simulink model "Control_RawPitchYaw"  (R2015b)
settings: Solver=FixedStepDiscrete  StartTime=0.0  StopTime=inf  FixedStep=0.03  RelTol=1e-3
undefined symbols (not defined in the file): DiscIntNeverNeededParam
libraries: simulink x7, arduinolib x4, RASPlib x2
settings Model: SimulationMode=external  ExtModeTrigDuration=2  Creator=jorge  LastModifiedBy=Emilio
settings OptimizationCC: OptimizeModelRefInitCode=on  LifeSpan=Inf  MaxStackSize=64
settings HardwareCC: ProdBitPerInt=16  ProdBitPerPointer=16  ProdLargestAtomicFloat=None  ProdWordSize=8  ProdHWDeviceType=Atmel->AVR
settings RTWCC: SystemTargetFile=ert.tlc  TemplateMakefile=ert_default_tmf  Description=Embedded Coder  Toolchain=Arduino AVR v1.6.1  BuildConfiguration=Faster Runs
settings CodeAppCC: IgnoreCustomStorageClasses=off
settings ERTTargetCC: SupportContinuousTime=on  SupportVariableSizeSignals=on  ExtMode=on  ExtModeMexFile=ext_serial_win32_comm_rtt  ExtModeMexArgs=0 5 115200

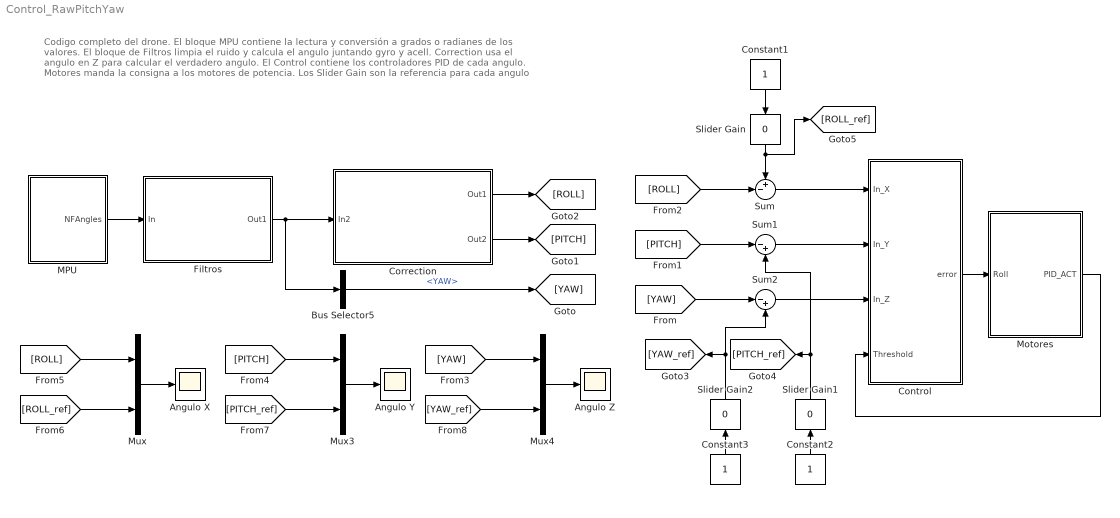
== system Control_RawPitchYaw ==
  note: Codigo completo del drone.
      | El bloque MPU contiene la lectura y conversión a grados o radianes de los valores.
      | El bloque de Filtros limpia el ruido y calcula el angulo juntando gyro y acell.
      | Correction usa el angulo en Z para calcular el verdadero angulo.
      | El Control contiene los controladores PID de cada angulo.
      | Motores manda la consigna a los motores de potencia.
      | Los Slider Gain son la referencia para cada angulo
  Angulo X : Scope
  Angulo Y : Scope
  Angulo Z : Scope
  Bus Selector5 : BusSelector  OutputSignals=YAW
  Constant1 : Constant
  Constant2 : Constant
  Constant3 : Constant
  Control : Subsystem
  Correction : Subsystem
  Filtros : Subsystem
  "MPU " : Subsystem
  "Motores " : Subsystem
  Mux : Mux  Inputs=2
  Mux3 : Mux  Inputs=2
  Mux4 : Mux  Inputs=2
  Slider Gain : simulink/Math Operations/Slider Gain  low=-25  gain=0  high=35
  Slider Gain1 : simulink/Math Operations/Slider Gain  low=-25  gain=0  high=35
  Slider Gain2 : simulink/Math Operations/Slider Gain  low=-25  gain=0  high=35
  Sum : Sum  Inputs=+-|
  Sum1 : Sum  Inputs=|-+
  Sum2 : Sum  Inputs=|-+
  wires:
  Mux/1 -> Angulo X/1
  Constant1/1 -> Slider Gain/1
  Slider Gain/1 -> Sum/1, [ROLL_ref]
  Constant2/1 -> Slider Gain1/1
  Sum/1 -> Control/1(In_X)
  Sum1/1 -> Control/2(In_Y)
  "Motores "/1(PID_ACT) -> Control/4(Threshold)
  Constant3/1 -> Slider Gain2/1
  Slider Gain2/1 -> Sum2/2, [YAW_ref]
  Sum2/1 -> Control/3(In_Z)
  Filtros/1(Out1) -> Bus Selector5/1, Correction/1(In2)
  "MPU "/1(NFAngles) -> Filtros/1(In)
  Bus Selector5/1 -> [YAW]  "<YAW>"
  Correction/2(Out2) -> [PITCH]
  Correction/1(Out1) -> [ROLL]
  [YAW] -> Sum2/1
  [PITCH] -> Sum1/1
  [ROLL] -> Sum/2
  Slider Gain1/1 -> [PITCH_ref], Sum1/2
  [ROLL] -> Mux/1
  [ROLL_ref] -> Mux/2
  [PITCH] -> Mux3/1
  [YAW] -> Mux4/1
  Mux3/1 -> Angulo Y/1
  Mux4/1 -> Angulo Z/1
  [PITCH_ref] -> Mux3/2
  [YAW_ref] -> Mux4/2
  Control/1(error) -> "Motores "/1(Roll)

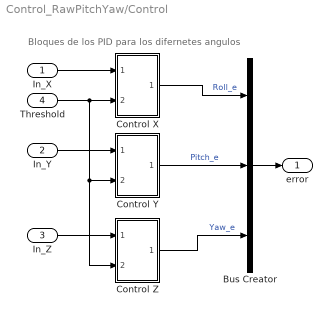
== system Control_RawPitchYaw/Control ==
  note: Bloques de los PID para los difernetes angulos
  In_X : Inport
  In_Y : Inport  Port=2
  In_Z : Inport  Port=3
  Threshold : Inport  Port=4
  Bus Creator : BusCreator  Inputs=3
  Control X : Subsystem
  Control Y : Subsystem
  Control Z : Subsystem
  error : Outport
  wires:
  Control X/1(Out1) -> Bus Creator/1  "Roll_e"
  Control Y/1(Out1) -> Bus Creator/2  "Pitch_e"
  In_Y/1 -> Control Y/1(In1)
  In_X/1 -> Control X/1(In1)
  In_Z/1 -> Control Z/1(In1)
  Threshold/1 -> Control Z/2(Threshold), Control Y/2(Threshold), Control X/2(Threshold)
  Control Z/1(Out1) -> Bus Creator/3  "Yaw_e"
  Bus Creator/1 -> error/1

== system Control_RawPitchYaw/Correction ==
  In2 : Inport
  Bus Selector3 : BusSelector  OutputSignals=NCAngle_X,NCAngle_y,Angle_Zrad
  Bus Selector4 : BusSelector  OutputSignals=NCAngle_y,NCAngle_X,Angle_Zrad
  CorrectionPITCH : Subsystem
  CorrectionROLL : Subsystem
  Out1 : Outport
  Out2 : Outport  Port=2
  wires:
  In2/1 -> Bus Selector3/1, Bus Selector4/1
  Bus Selector4/2 -> CorrectionPITCH/2(Angle_Corr)  "<NCAngle_X>"
  Bus Selector3/1 -> CorrectionROLL/1(Angle_cal)  "<NCAngle_X>"
  Bus Selector3/3 -> CorrectionROLL/3(Z_Corr)  "<Angle_Zrad>"
  Bus Selector4/1 -> CorrectionPITCH/1(Angle_cal)  "<NCAngle_y>"
  Bus Selector3/2 -> CorrectionROLL/2(Angle_Corr)  "<NCAngle_y>"
  Bus Selector4/3 -> CorrectionPITCH/3(Z_Corr)  "<Angle_Zrad>"
  CorrectionPITCH/1(Angle_Corrected) -> Out2/1  "PITCH"
  CorrectionROLL/1(Angle_Corrected) -> Out1/1  "ROLL"

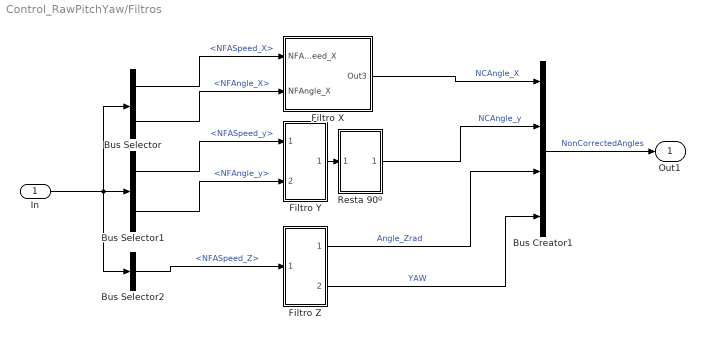
== system Control_RawPitchYaw/Filtros ==
  In : Inport
  Bus Creator1 : BusCreator  Inputs=4
  Bus Selector : BusSelector  OutputSignals=NFASpeed_X,NFAngle_X
  Bus Selector1 : BusSelector  OutputSignals=NFASpeed_y,NFAngle_y
  Bus Selector2 : BusSelector  OutputSignals=NFASpeed_Z
  Filtro X : Subsystem
  Filtro Y : Subsystem
  "Filtro Z " : Subsystem
  Resta 90º : Subsystem
  Out1 : Outport
  wires:
  Bus Creator1/1 -> Out1/1  "NonCorrectedAngles"
  Filtro X/1(Out3) -> Bus Creator1/1  "NCAngle_X"
  Bus Selector/1 -> Filtro X/1(NFASpeed_X)  "<NFASpeed_X>"
  Bus Selector2/1 -> "Filtro Z "/1(In1)  "<NFASpeed_Z>"
  Bus Selector1/1 -> Filtro Y/1(In1)  "<NFASpeed_y>"
  Bus Selector/2 -> Filtro X/2(NFAngle_X)  "<NFAngle_X>"
  Bus Selector1/2 -> Filtro Y/2(In2)  "<NFAngle_y>"
  In/1 -> Bus Selector/1, Bus Selector2/1, Bus Selector1/1
  Resta 90º/1(Out1) -> Bus Creator1/2  "NCAngle_y"
  "Filtro Z "/1(Z radianes) -> Bus Creator1/3  "Angle_Zrad"
  Filtro Y/1(Out3) -> Resta 90º/1(In1)
  "Filtro Z "/2(Z grados) -> Bus Creator1/4  "YAW"

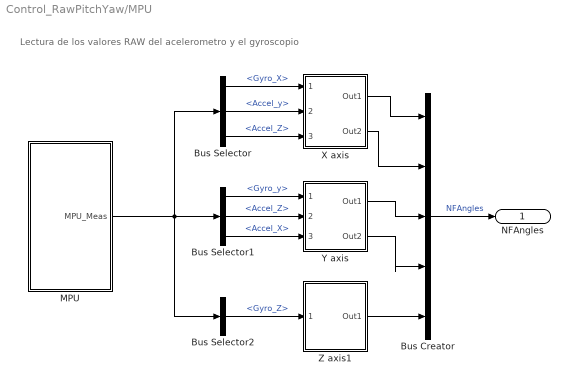
== system Control_RawPitchYaw/MPU  ==
  note: Lectura de los valores RAW del acelerometro y el gyroscopio
  Bus Creator : BusCreator  Inputs='NFASpeed_X','NFAngle_X','NFASpeed_y','NFAngle_y','NFASpeed_Z'
  Bus Selector : BusSelector  OutputSignals=Gyro_X,Accel_y,Accel_Z
  Bus Selector1 : BusSelector  OutputSignals=Gyro_y,Accel_Z,Accel_X
  Bus Selector2 : BusSelector  OutputSignals=Gyro_Z
  MPU : Subsystem
  X axis : Subsystem
  Y axis : Subsystem
  Z axis1 : Subsystem
  NFAngles : Outport
  wires:
  MPU/1(MPU_Meas) -> Bus Selector/1, Bus Selector1/1, Bus Selector2/1
  Bus Selector/2 -> X axis/2(Accel_y)  "<Accel_y>"
  Bus Selector/3 -> X axis/3(Accel_Z)  "<Accel_Z>"
  Bus Selector/1 -> X axis/1(Gyro_X)  "<Gyro_X>"
  Bus Selector1/2 -> Y axis/2(Accel_Z)  "<Accel_Z>"
  Bus Selector1/3 -> Y axis/3(Accel_X)  "<Accel_X>"
  Bus Selector1/1 -> Y axis/1(Gyro_y)  "<Gyro_y>"
  Bus Selector2/1 -> Z axis1/1(Gyro_Z)  "<Gyro_Z>"
  Bus Creator/1 -> NFAngles/1  "NFAngles"
  X axis/1(Out1) -> Bus Creator/1
  X axis/2(Out2) -> Bus Creator/2
  Y axis/1(Out1) -> Bus Creator/3
  Y axis/2(Out2) -> Bus Creator/4
  Z axis1/1(Out1) -> Bus Creator/5

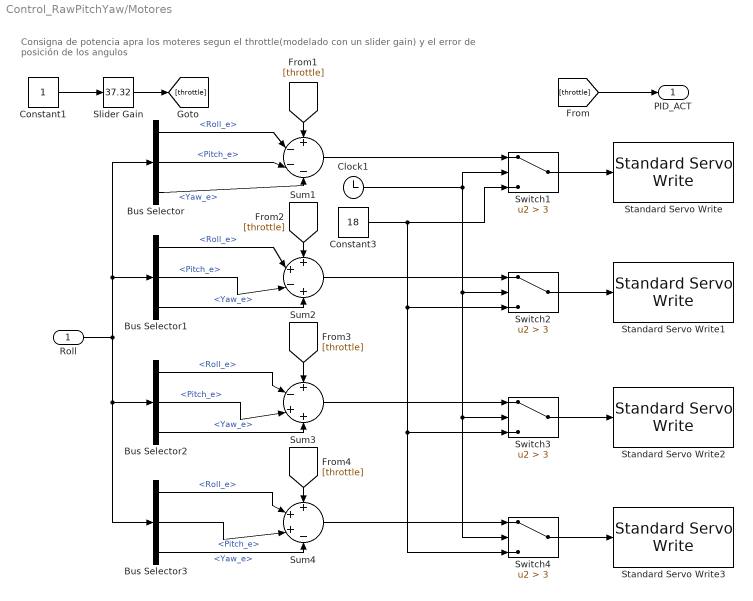
== system Control_RawPitchYaw/Motores  ==
  note: Consigna de potencia apra los moteres segun el throttle(modelado con un slider gain) y el error de posición de los angulos
  Roll : Inport
  Bus Selector{,1..3} (4 alike) : BusSelector  OutputSignals=Roll_e,Pitch_e,Yaw_e
  Clock1 : Clock
  Constant1 : Constant
  Constant3 : Constant  Value=18
  Slider Gain : simulink/Math Operations/Slider Gain  low=18  gain=37.32  high=60
  Standard Servo Write : arduinolib/Standard Servo Write  pinNumber=12  blockPlatform=arduino
  Standard Servo Write1 : arduinolib/Standard Servo Write  pinNumber=11  blockPlatform=arduino
  Standard Servo Write2 : arduinolib/Standard Servo Write  pinNumber=10  blockPlatform=arduino
  Standard Servo Write3 : arduinolib/Standard Servo Write  pinNumber=9  blockPlatform=arduino
  Sum1 : Sum  Inputs=+|-|-|-
  Sum2 : Sum  Inputs=+|+|-|+
  Sum3 : Sum  Inputs=+|-|+|+
  Sum4 : Sum  Inputs=+|+|+|-
  Switch{1..4} (4 alike) : Switch  Criteria=u2 > Threshold  Threshold=3
  PID_ACT : Outport
  wires:
  Constant3/1 -> Switch4/3, Switch3/3, Switch2/3, Switch1/3
  Sum4/1 -> Switch4/1
  Clock1/1 -> Switch1/2, Switch4/2, Switch3/2, Switch2/2
  Sum3/1 -> Switch3/1
  Switch4/1 -> Standard Servo Write3/1
  Switch3/1 -> Standard Servo Write2/1
  Sum1/1 -> Switch1/1
  Switch1/1 -> Standard Servo Write/1
  Switch2/1 -> Standard Servo Write1/1
  Sum2/1 -> Switch2/1
  Constant1/1 -> Slider Gain/1
  Roll/1 -> Bus Selector3/1, Bus Selector2/1, Bus Selector/1, Bus Selector1/1
  Bus Selector/1 -> Sum1/2  "<Roll_e>"
  Bus Selector/2 -> Sum1/3  "<Pitch_e>"
  Bus Selector/3 -> Sum1/4  "<Yaw_e>"
  Bus Selector1/1 -> Sum2/2  "<Roll_e>"
  Bus Selector1/2 -> Sum2/3  "<Pitch_e>"
  Bus Selector1/3 -> Sum2/4  "<Yaw_e>"
  Bus Selector2/1 -> Sum3/2  "<Roll_e>"
  Bus Selector2/2 -> Sum3/3  "<Pitch_e>"
  Bus Selector2/3 -> Sum3/4  "<Yaw_e>"
  Bus Selector3/1 -> Sum4/2  "<Roll_e>"
  Bus Selector3/2 -> Sum4/3  "<Pitch_e>"
  Bus Selector3/3 -> Sum4/4  "<Yaw_e>"
  Slider Gain/1 -> [throttle]
  [throttle] -> PID_ACT/1
  [throttle] -> Sum1/1
  [throttle] -> Sum2/1
  [throttle] -> Sum3/1
  [throttle] -> Sum4/1

== system Control_RawPitchYaw/Control/Control X ==
  note: PID con un threshold apra evitar que el integrador acumule antes que el control pueda mover el drone
  In1 : Inport
  Threshold : Inport  Port=2
  Constant2 : Constant  Value=0
  Discrete PID Controller : simulink/Continuous/PID Controller  Controller=PID  TimeDomain=Discrete-time  SampleTime=-1  IntegratorMethod=Forward Euler  FilterMethod=Forward Euler  Form=Parallel  UseFilter=off  ControllerParametersSource=internal  P=0.51  I=0.43  D=0.15  N=30  InitialConditionSource=internal  InitialConditionForIntegrator=0  InitialConditionForFilter=0  ExternalReset=rising  LimitOutput=off  UpperSaturationLimit=inf  LowerSaturationLimit=-inf  LinearizeAsGain=off  AntiWindupMode=none  Kb=1  TrackingMode=off  Kt=1  PParamMin=[]  PParamMax=[]  IParamMin=[]  IParamMax=[]  DParamMin=[]  DParamMax=[]  NParamMin=[]  NParamMax=[]  KbParamMin=[]  KbParamMax=[]  KtParamMin=[]  KtParamMax=[]  POutMin=[]  POutMax=[]  IOutMin=[]  IOutMax=[]  DOutMin=[]  DOutMax=[]  NOutMin=[]  NOutMax=[]  KbOutMin=[]  KbOutMax=[]  KtOutMin=[]  KtOutMax=[]  IntegratorOutMin=[]  IntegratorOutMax=[]  FilterOutMin=[]  FilterOutMax=[]  SumOutMin=[]  SumOutMax=[]  SumI1OutMin=[]  SumI1OutMax=[]  SumI2OutMin=[]  SumI2OutMax=[]  SumI3OutMin=[]  SumI3OutMax=[]  SumDOutMin=[]  SumDOutMax=[]  SaturationOutMin=[]  SaturationOutMax=[]  IntegratorContinuousStateAttributes=''  IntegratorStateMustResolveToSignalObject=off  IntegratorRTWStateStorageClass=Auto  FilterContinuousStateAttributes=''  FilterStateMustResolveToSignalObject=off  FilterRTWStateStorageClass=Auto  DifferentiatorICPrevScaledInput=0  DifferentiatorOutMin=[]  DifferentiatorOutMax=[]
  Pulse Generator : DiscretePulseGenerator  Commented=on  Period=167  PulseWidth=5  SampleTime=0.03
  Switch1 : Switch  Criteria=u2 > Threshold  Threshold=35
  Out1 : Outport
  wires:
  Discrete PID Controller/1 -> Out1/1
  Switch1/1 -> Discrete PID Controller/1
  Threshold/1 -> Switch1/2
  Constant2/1 -> Switch1/3
  In1/1 -> Switch1/1
  Pulse Generator/1 -> Discrete PID Controller/2

== system Control_RawPitchYaw/Control/Control Y ==
  In1 : Inport
  Threshold : Inport  Port=2
  Constant2 : Constant  Value=0
  Discrete PID Controller : simulink/Continuous/PID Controller  Controller=PID  TimeDomain=Discrete-time  SampleTime=-1  IntegratorMethod=Forward Euler  FilterMethod=Forward Euler  Form=Parallel  UseFilter=off  ControllerParametersSource=internal  P=0.51  I=0.43  D=0.15  N=30  InitialConditionSource=internal  InitialConditionForIntegrator=0  InitialConditionForFilter=0  ExternalReset=rising  LimitOutput=off  UpperSaturationLimit=inf  LowerSaturationLimit=-inf  LinearizeAsGain=off  AntiWindupMode=none  Kb=1  TrackingMode=off  Kt=1  PParamMin=[]  PParamMax=[]  IParamMin=[]  IParamMax=[]  DParamMin=[]  DParamMax=[]  NParamMin=[]  NParamMax=[]  KbParamMin=[]  KbParamMax=[]  KtParamMin=[]  KtParamMax=[]  POutMin=[]  POutMax=[]  IOutMin=[]  IOutMax=[]  DOutMin=[]  DOutMax=[]  NOutMin=[]  NOutMax=[]  KbOutMin=[]  KbOutMax=[]  KtOutMin=[]  KtOutMax=[]  IntegratorOutMin=[]  IntegratorOutMax=[]  FilterOutMin=[]  FilterOutMax=[]  SumOutMin=[]  SumOutMax=[]  SumI1OutMin=[]  SumI1OutMax=[]  SumI2OutMin=[]  SumI2OutMax=[]  SumI3OutMin=[]  SumI3OutMax=[]  SumDOutMin=[]  SumDOutMax=[]  SaturationOutMin=[]  SaturationOutMax=[]  IntegratorContinuousStateAttributes=''  IntegratorStateMustResolveToSignalObject=off  IntegratorRTWStateStorageClass=Auto  FilterContinuousStateAttributes=''  FilterStateMustResolveToSignalObject=off  FilterRTWStateStorageClass=Auto  DifferentiatorICPrevScaledInput=0  DifferentiatorOutMin=[]  DifferentiatorOutMax=[]
  Pulse Generator : DiscretePulseGenerator  Commented=on  Period=167  PulseWidth=5  SampleTime=0.03
  Switch1 : Switch  Criteria=u2 > Threshold  Threshold=35
  Out1 : Outport
  wires:
  Discrete PID Controller/1 -> Out1/1
  Switch1/1 -> Discrete PID Controller/1
  Threshold/1 -> Switch1/2
  Constant2/1 -> Switch1/3
  In1/1 -> Switch1/1
  Pulse Generator/1 -> Discrete PID Controller/2

== system Control_RawPitchYaw/Control/Control Z ==
  In1 : Inport
  Threshold : Inport  Port=2
  Constant2 : Constant  Value=0
  Discrete PID Controller : simulink/Continuous/PID Controller  Controller=PID  TimeDomain=Discrete-time  SampleTime=-1  IntegratorMethod=Forward Euler  FilterMethod=Forward Euler  Form=Parallel  UseFilter=off  ControllerParametersSource=internal  P=0.1  I=0  D=0  N=30  InitialConditionSource=internal  InitialConditionForIntegrator=0  InitialConditionForFilter=0  ExternalReset=rising  LimitOutput=off  UpperSaturationLimit=inf  LowerSaturationLimit=-inf  LinearizeAsGain=off  AntiWindupMode=none  Kb=1  TrackingMode=off  Kt=1  PParamMin=[]  PParamMax=[]  IParamMin=[]  IParamMax=[]  DParamMin=[]  DParamMax=[]  NParamMin=[]  NParamMax=[]  KbParamMin=[]  KbParamMax=[]  KtParamMin=[]  KtParamMax=[]  POutMin=[]  POutMax=[]  IOutMin=[]  IOutMax=[]  DOutMin=[]  DOutMax=[]  NOutMin=[]  NOutMax=[]  KbOutMin=[]  KbOutMax=[]  KtOutMin=[]  KtOutMax=[]  IntegratorOutMin=[]  IntegratorOutMax=[]  FilterOutMin=[]  FilterOutMax=[]  SumOutMin=[]  SumOutMax=[]  SumI1OutMin=[]  SumI1OutMax=[]  SumI2OutMin=[]  SumI2OutMax=[]  SumI3OutMin=[]  SumI3OutMax=[]  SumDOutMin=[]  SumDOutMax=[]  SaturationOutMin=[]  SaturationOutMax=[]  IntegratorContinuousStateAttributes=''  IntegratorStateMustResolveToSignalObject=off  IntegratorRTWStateStorageClass=Auto  FilterContinuousStateAttributes=''  FilterStateMustResolveToSignalObject=off  FilterRTWStateStorageClass=Auto  DifferentiatorICPrevScaledInput=0  DifferentiatorOutMin=[]  DifferentiatorOutMax=[]
  Pulse Generator : DiscretePulseGenerator  Commented=on  Period=167  PulseWidth=5  SampleTime=0.03
  Switch1 : Switch  Criteria=u2 > Threshold  Threshold=25
  Out1 : Outport
  wires:
  Discrete PID Controller/1 -> Out1/1
  Switch1/1 -> Discrete PID Controller/1
  Threshold/1 -> Switch1/2
  Constant2/1 -> Switch1/3
  In1/1 -> Switch1/1
  Pulse Generator/1 -> Discrete PID Controller/2

== system Control_RawPitchYaw/Correction/CorrectionPITCH ==
  note: Correción al angulo usando las medidas en Z
  Angle_cal : Inport
  Angle_Corr : Inport  Port=2
  Z_Corr : Inport  Port=3
  Product : Product
  Sum2 : Sum  Inputs=++|
  Trigonometric Function : Trigonometry
  Angle_Corrected : Outport
  wires:
  Angle_Corr/1 -> Product/1
  Sum2/1 -> Angle_Corrected/1
  Z_Corr/1 -> Trigonometric Function/1
  Angle_cal/1 -> Sum2/1
  Product/1 -> Sum2/2
  Trigonometric Function/1 -> Product/2

== system Control_RawPitchYaw/Correction/CorrectionROLL ==
  note: Correción al angulo usando las medidas en Z
  Angle_cal : Inport
  Angle_Corr : Inport  Port=2
  Z_Corr : Inport  Port=3
  Product : Product
  Sum2 : Sum  Inputs=++|
  Trigonometric Function : Trigonometry
  Angle_Corrected : Outport
  wires:
  Trigonometric Function/1 -> Product/2
  Product/1 -> Sum2/2
  Angle_cal/1 -> Sum2/1
  Z_Corr/1 -> Trigonometric Function/1
  Sum2/1 -> Angle_Corrected/1
  Angle_Corr/1 -> Product/1

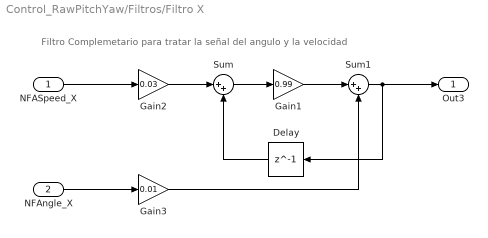
== system Control_RawPitchYaw/Filtros/Filtro X ==
  note: Filtro Complemetario para tratar la señal del angulo y la velocidad
  NFASpeed_X : Inport
  NFAngle_X : Inport  Port=2
  Delay : Delay  DelayLength=1  InitialCondition=0
  Gain1 : Gain  Gain=0.99
  Gain2 : Gain  Gain=0.03
  Gain3 : Gain  Gain=0.01
  Sum : Sum  Inputs=|++
  Sum1 : Sum  Inputs=|++
  Out3 : Outport
  wires:
  Delay/1 -> Sum/2
  Sum/1 -> Gain1/1
  NFAngle_X/1 -> Gain3/1
  Gain1/1 -> Sum1/1
  Sum1/1 -> Out3/1, Delay/1
  NFASpeed_X/1 -> Gain2/1
  Gain2/1 -> Sum/1
  Gain3/1 -> Sum1/2

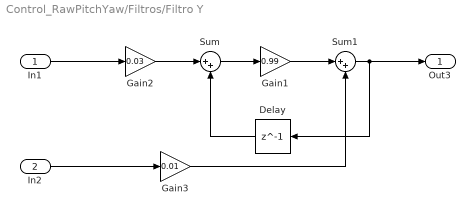
== system Control_RawPitchYaw/Filtros/Filtro Y ==
  In1 : Inport
  In2 : Inport  Port=2
  Delay : Delay  DelayLength=1  InitialCondition=0
  Gain1 : Gain  Gain=0.99
  Gain2 : Gain  Gain=0.03
  Gain3 : Gain  Gain=0.01
  Sum : Sum  Inputs=|++
  Sum1 : Sum  Inputs=|++
  Out3 : Outport
  wires:
  Delay/1 -> Sum/2
  Sum/1 -> Gain1/1
  In2/1 -> Gain3/1
  Gain1/1 -> Sum1/1
  Sum1/1 -> Out3/1, Delay/1
  In1/1 -> Gain2/1
  Gain2/1 -> Sum/1
  Gain3/1 -> Sum1/2

== system Control_RawPitchYaw/Filtros/Filtro Z  ==
  note: Integración de la velocidad en Z para sacar el angulo en radianes y grados
  In1 : Inport
  Discrete-Time Integrator : DiscreteIntegrator  InitialConditionSetting=State (most efficient)  SampleTime=-1  ICPrevOutput=DiscIntNeverNeededParam  ICPrevScaledInput=DiscIntNeverNeededParam
  Gain : Gain  Gain=3.1416/180
  Z radianes : Outport
  Z grados : Outport  Port=2
  wires:
  In1/1 -> Discrete-Time Integrator/1
  Gain/1 -> Z radianes/1
  Discrete-Time Integrator/1 -> Z grados/1, Gain/1

== system Control_RawPitchYaw/Filtros/Resta 90º ==
  In1 : Inport
  Add : Sum  Inputs=+-
  resta90º : Constant  Value=90
  Out1 : Outport
  wires:
  resta90º/1 -> Add/2
  In1/1 -> Add/1
  Add/1 -> Out1/1

== system Control_RawPitchYaw/MPU /MPU ==
  note: Valores RAW de los sensores
  Accelerometer : RASPlib/Accelerometer  SimulateUsing=Code generation
  Bus Creator : BusCreator  Inputs='Gyro_X','Gyro_y','Gyro_Z','Accel_X','Accel_y','Accel_Z'
  Gyroscope : RASPlib/Gyroscope  DLPFmode=0
  MPU_Meas : Outport
  wires:
  Accelerometer/3 -> Bus Creator/6  "Accel_Z"
  Gyroscope/3 -> Bus Creator/3  "Gyro_Z"
  Accelerometer/2 -> Bus Creator/5  "Accel_y"
  Gyroscope/2 -> Bus Creator/2  "Gyro_y"
  Accelerometer/1 -> Bus Creator/4  "Accel_X"
  Bus Creator/1 -> MPU_Meas/1  "MPU_meas"
  Gyroscope/1 -> Bus Creator/1  "Gyro_X"

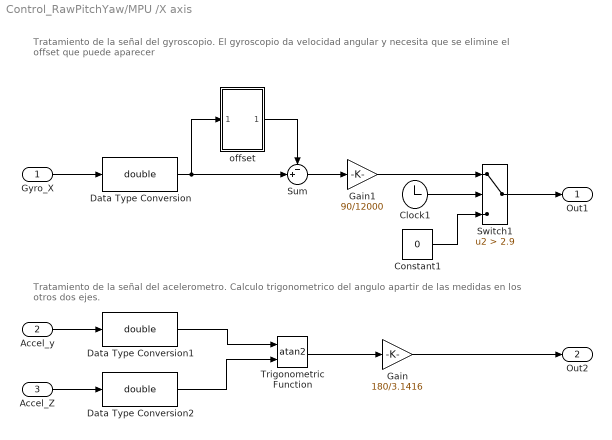
== system Control_RawPitchYaw/MPU /X axis ==
  note: Tratamiento de la señal del acelerometro.
      | Calculo trigonometrico del angulo apartir de las medidas en los otros dos ejes.
  note: Tratamiento de la señal del gyroscopio.
      | El gyroscopio da velocidad angular y necesita que se elimine el offset que puede aparecer
  Gyro_X : Inport
  Accel_y : Inport  Port=2
  Accel_Z : Inport  Port=3
  Clock1 : Clock
  Constant1 : Constant  Value=0
  Data Type Conversion : DataTypeConversion  OutDataTypeStr=double
  Data Type Conversion1 : DataTypeConversion  OutDataTypeStr=double
  Data Type Conversion2 : DataTypeConversion  OutDataTypeStr=double
  Gain : Gain  Gain=180/3.1416
  Gain1 : Gain  Gain=90/12000
  Sum : Sum  Inputs=-+|
  Switch1 : Switch  Criteria=u2 > Threshold  Threshold=2.9
  Trigonometric Function : Trigonometry  Operator=atan2
  offset : Subsystem
  Out1 : Outport
  Out2 : Outport  Port=2
  wires:
  Sum/1 -> Gain1/1
  Gain/1 -> Out2/1
  Clock1/1 -> Switch1/2
  Trigonometric Function/1 -> Gain/1
  Data Type Conversion/1 -> offset/1(In1), Sum/2
  Switch1/1 -> Out1/1
  Data Type Conversion1/1 -> Trigonometric Function/1
  Data Type Conversion2/1 -> Trigonometric Function/2
  Accel_y/1 -> Data Type Conversion1/1
  Constant1/1 -> Switch1/3
  Accel_Z/1 -> Data Type Conversion2/1
  Gyro_X/1 -> Data Type Conversion/1
  Gain1/1 -> Switch1/1
  offset/1(Out1) -> Sum/1

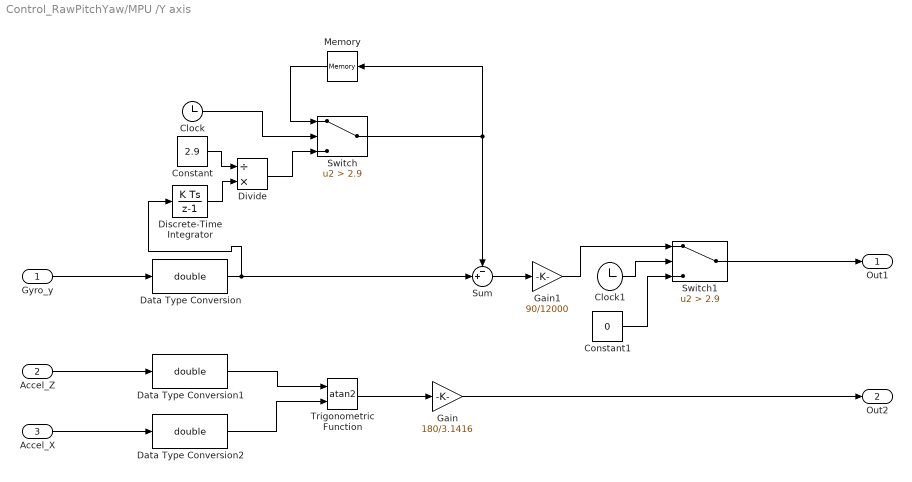
== system Control_RawPitchYaw/MPU /Y axis ==
  Gyro_y : Inport
  Accel_Z : Inport  Port=2
  Accel_X : Inport  Port=3
  Clock : Clock
  Clock1 : Clock
  Constant : Constant  Value=2.9
  Constant1 : Constant  Value=0
  Data Type Conversion : DataTypeConversion  OutDataTypeStr=double
  Data Type Conversion1 : DataTypeConversion  OutDataTypeStr=double
  Data Type Conversion2 : DataTypeConversion  OutDataTypeStr=double
  Discrete-Time Integrator : DiscreteIntegrator  InitialConditionSetting=State (most efficient)  SampleTime=-1  ICPrevOutput=DiscIntNeverNeededParam  ICPrevScaledInput=DiscIntNeverNeededParam
  Divide : Product  Inputs=/*
  Gain : Gain  Gain=180/3.1416
  Gain1 : Gain  Gain=90/12000
  Memory : Memory
  Sum : Sum  Inputs=-+|
  Switch : Switch  Criteria=u2 > Threshold  Threshold=2.9
  Switch1 : Switch  Criteria=u2 > Threshold  Threshold=2.9
  Trigonometric Function : Trigonometry  Operator=atan2
  Out1 : Outport
  Out2 : Outport  Port=2
  wires:
  Sum/1 -> Gain1/1
  Clock/1 -> Switch/2
  Switch/1 -> Sum/1, Memory/1
  Constant/1 -> Divide/1
  Gain/1 -> Out2/1
  Clock1/1 -> Switch1/2
  Trigonometric Function/1 -> Gain/1
  Data Type Conversion/1 -> Sum/2, Discrete-Time Integrator/1
  Switch1/1 -> Out1/1
  Data Type Conversion1/1 -> Trigonometric Function/1
  Data Type Conversion2/1 -> Trigonometric Function/2
  Accel_Z/1 -> Data Type Conversion1/1
  Constant1/1 -> Switch1/3
  Accel_X/1 -> Data Type Conversion2/1
  Divide/1 -> Switch/3
  Memory/1 -> Switch/1
  Discrete-Time Integrator/1 -> Divide/2
  Gyro_y/1 -> Data Type Conversion/1
  Gain1/1 -> Switch1/1

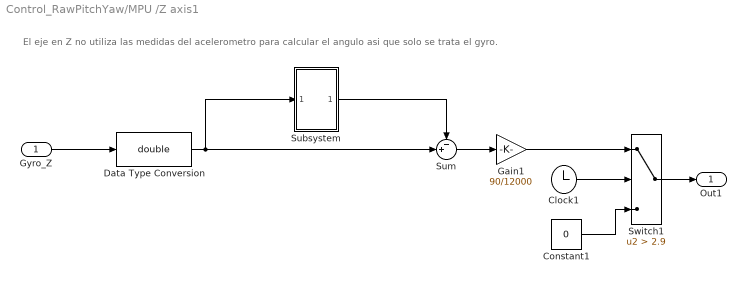
== system Control_RawPitchYaw/MPU /Z axis1 ==
  note: El eje en Z no utiliza las medidas del acelerometro para calcular el angulo asi que solo se trata el gyro.
  Gyro_Z : Inport
  Clock1 : Clock
  Constant1 : Constant  Value=0
  Data Type Conversion : DataTypeConversion  OutDataTypeStr=double
  Gain1 : Gain  Gain=90/12000
  Subsystem : Subsystem
  Sum : Sum  Inputs=-+|
  Switch1 : Switch  Criteria=u2 > Threshold  Threshold=2.9
  Out1 : Outport
  wires:
  Sum/1 -> Gain1/1
  Clock1/1 -> Switch1/2
  Data Type Conversion/1 -> Subsystem/1(In1), Sum/2
  Switch1/1 -> Out1/1
  Constant1/1 -> Switch1/3
  Gyro_Z/1 -> Data Type Conversion/1
  Gain1/1 -> Switch1/1
  Subsystem/1(Out1) -> Sum/1

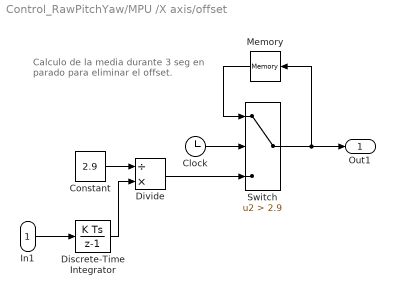
== system Control_RawPitchYaw/MPU /X axis/offset ==
  note: Calculo de la media durante 3 seg en parado para eliminar el offset.
  In1 : Inport
  Clock : Clock
  Constant : Constant  Value=2.9
  Discrete-Time Integrator : DiscreteIntegrator  InitialConditionSetting=State (most efficient)  SampleTime=-1  ICPrevOutput=DiscIntNeverNeededParam  ICPrevScaledInput=DiscIntNeverNeededParam
  Divide : Product  Inputs=/*
  Memory : Memory
  Switch : Switch  Criteria=u2 > Threshold  Threshold=2.9
  Out1 : Outport
  wires:
  Switch/1 -> Out1/1, Memory/1
  Discrete-Time Integrator/1 -> Divide/2
  Divide/1 -> Switch/3
  Memory/1 -> Switch/1
  Clock/1 -> Switch/2
  Constant/1 -> Divide/1
  In1/1 -> Discrete-Time Integrator/1

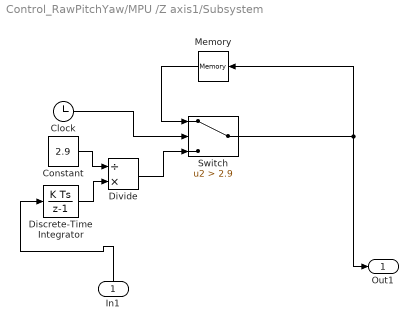
== system Control_RawPitchYaw/MPU /Z axis1/Subsystem ==
  In1 : Inport
  Clock : Clock
  Constant : Constant  Value=2.9
  Discrete-Time Integrator : DiscreteIntegrator  InitialConditionSetting=State (most efficient)  SampleTime=-1  ICPrevOutput=DiscIntNeverNeededParam  ICPrevScaledInput=DiscIntNeverNeededParam
  Divide : Product  Inputs=/*
  Memory : Memory
  Switch : Switch  Criteria=u2 > Threshold  Threshold=2.9
  Out1 : Outport
  wires:
  Switch/1 -> Out1/1, Memory/1
  Divide/1 -> Switch/3
  Clock/1 -> Switch/2
  Memory/1 -> Switch/1
  Discrete-Time Integrator/1 -> Divide/2
  Constant/1 -> Divide/1
  In1/1 -> Discrete-Time Integrator/1
